simulink model "mix"  (R2018b)
settings: Solver=VariableStepAuto  StartTime=0.0  StopTime=10  RelTol=1e-3
values from neighbouring files (symbols this model uses):
  A = [0,1,0,0;-ks/Il,-cl/Il,ks/Il,0;0,0,0,1;ks/Im,0,-ks/Im,-cm/Im]    [base_mix.m]    (also in optimal_control.m)
  B = [0,0;0,1/Il;0,0;K/Im,0]    [base_mix.m]    (also in optimal_control.m)
  C = [0,0,1,0;1,0,0,0;-ks,0,ks,0]    [base_mix.m]    (also in optimal_control.m)
  D = zeros(3,2)    [base_mix.m]    (also in optimal_control.m)
  G = G(4)    [base_mix.m]    (also in optimal_control.m)
  Kd = (2*ksai_torque*wn_torque+beta_torque)/den    [base_mix.m]
  Kf = acker(A,B(:,1),Target_Pole)    [base_mix.m]    (also in optimal_control.m = lqr(A,B(:,1),Q,R))
  Ki = (beta_torque*wn_torque^2)/den    [base_mix.m]
  Kp = ((2*ksai_torque*wn_torque*beta_torque+wn_torque^2-(Il+Im)*ks/Il/Im))/den    [base_mix.m]
libraries: cstblocks x2, simulink x1
settings Model: Creator=78224  LastModifiedBy=78224

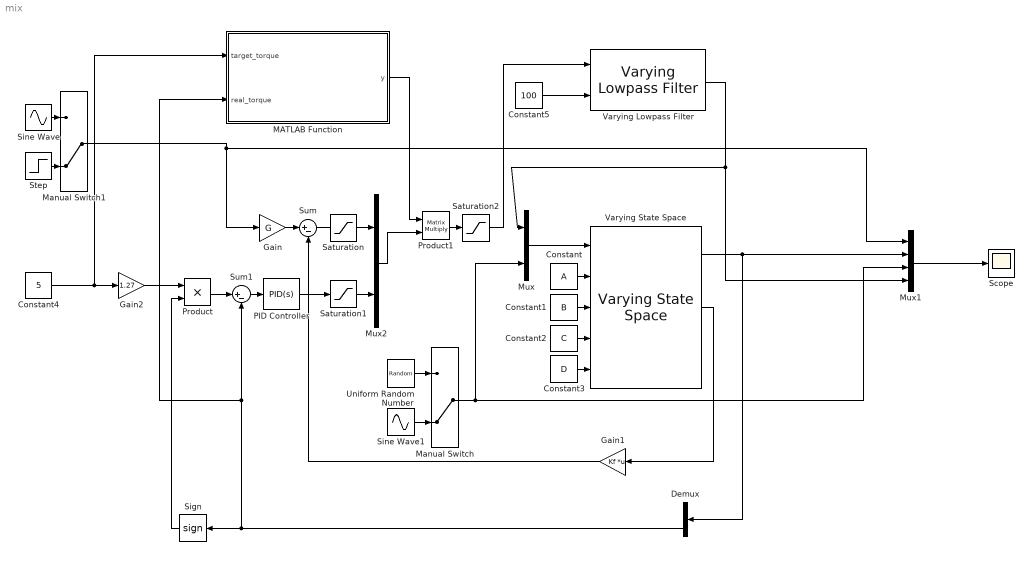
== system mix ==
  Constant : Constant  Value=A  VectorParams1D=off
  Constant1 : Constant  Value=B  VectorParams1D=off
  Constant2 : Constant  Value=C  VectorParams1D=off
  Constant3 : Constant  Value=D  VectorParams1D=off
  Constant4 : Constant  Value=5
  Constant5 : Constant  Value=100
  Demux : Demux  Outputs=3
  Gain : Gain  Gain=G
  Gain1 : Gain  Gain=Kf  Multiplication=Matrix(K*u)
  Gain2 : Gain  Gain=1.27
  MATLAB Function : MATLAB Function  TreatAsAtomicUnit=on
  Manual Switch : ManualSwitch  CurrentSetting=0
  Manual Switch1 : ManualSwitch  CurrentSetting=0
  Mux : Mux  Inputs=2
  Mux1 : Mux
  Mux2 : Mux  Inputs=2
  PID Controller : simulink/Continuous/PID Controller  Controller=PID  Form=Parallel  TimeDomain=Continuous-time  SampleTime=-1  IntegratorMethod=Forward Euler  FilterMethod=Forward Euler  ControllerParametersSource=internal  P=Kp  I=Ki  D=Kd  UseFilter=on  N=100  TunerSelectOption=Transfer Function Based (PID Tuner App)  InitialConditionSource=internal  InitialConditionForIntegrator=0  InitialConditionForFilter=0  DifferentiatorICPrevScaledInput=0  ExternalReset=none  TrackingMode=off  Kt=1  LimitOutput=off  UpperSaturationLimit=inf  LowerSaturationLimit=-inf  LinearizeAsGain=on  AntiWindupMode=none  Kb=1  POutMin=[]  POutMax=[]  IOutMin=[]  IOutMax=[]  DOutMin=[]  DOutMax=[]  NOutMin=[]  NOutMax=[]  SumOutMin=[]  SumOutMax=[]  SaturationOutMin=[]  SaturationOutMax=[]  PParamMin=[]  PParamMax=[]  IParamMin=[]  IParamMax=[]  DParamMin=[]  DParamMax=[]  NParamMin=[]  NParamMax=[]  KbParamMin=[]  KbParamMax=[]  KtParamMin=[]  KtParamMax=[]  KbOutMin=[]  KbOutMax=[]  KtOutMin=[]  KtOutMax=[]  IntegratorOutMin=[]  IntegratorOutMax=[]  FilterOutMin=[]  FilterOutMax=[]  SumI1OutMin=[]  SumI1OutMax=[]  SumI2OutMin=[]  SumI2OutMax=[]  SumI3OutMin=[]  SumI3OutMax=[]  SumI4OutMin=[]  SumI4OutMax=[]  SumDOutMin=[]  SumDOutMax=[]  DifferentiatorOutMin=[]  DifferentiatorOutMax=[]  FilterDiffOutCoefMin=[]  FilterDiffOutCoefMax=[]  ReciprocalOutMin=[]  ReciprocalOutMax=[]  SumDenOutMin=[]  SumDenOutMax=[]  SumNumOutMin=[]  SumNumOutMax=[]  DivideOutMin=[]  DivideOutMax=[]  IntegratorContinuousStateAttributes=''  IntegratorStateMustResolveToSignalObject=off  IntegratorRTWStateStorageClass=Auto  FilterContinuousStateAttributes=''  FilterStateMustResolveToSignalObject=off  FilterRTWStateStorageClass=Auto  ParallelPVariant=InternalParameters  IdealPVariant=Disabled  IVariant=InternalParameters  DVariant=InternalParameters  IntegratorVariant=Continuous  SatVariant=Disabled  AWVariant=Passthrough  PCopyVariant=Disabled  TRVariant=Disabled  FdbkBlocksVariant=Forward  IdealPFdbkVariant=Disabled  SatFdbkVariant=Disabled  DerivativeFilterVariant=ContFilter  NVariant=InternalParameters  NCopyVariant=Disabled  FilterICVariant=InternalICsFilter  IntegratorICVariant=InternalICs  ExternalResetVariant=Disabled  TRSumVariant=Passthrough  SumFdbkVariant=Disabled  SumVariant=Sum_PID
  Product : Product
  Product1 : Product  Multiplication=Matrix(*)
  Saturation : Saturate  UpperLimit=3.12  LowerLimit=-3.12
  Saturation1 : Saturate  UpperLimit=3.12  LowerLimit=-3.12
  Saturation2 : Saturate  UpperLimit=3.12  LowerLimit=-3.12
  Scope : Scope
  Sign : Signum
  Sine Wave : Sin  Amplitude=60  Frequency=2*pi*0.2  SampleTime=0
  Sine Wave1 : Sin  Amplitude=0  Frequency=2*pi*0.2  SampleTime=0
  Step : Step  After=60  SampleTime=0
  Sum : Sum  Inputs=|+-
  Sum1 : Sum  Inputs=|+-
  Uniform Random Number : UniformRandomNumber  Minimum=-5  Maximum=5  SampleTime=0.1
  Varying Lowpass Filter : cstblocks/Linear Parameter Varying/Varying Lowpass Filter  N=1
      settings: SourceProductName=Control System Toolbox
  Varying State Space : cstblocks/Linear Parameter Varying/Varying State Space  x0=0  xNames=''  OutputX=on  OutputDX=on
      settings: SourceProductName=Control System Toolbox
  wires:
  Saturation1/1 -> Mux2/2
  Varying Lowpass Filter/1 -> Mux1/4, Mux/1
  Mux2/1 -> Product1/2
  Step/1 -> Manual Switch1/2
  Sum/1 -> Mux2/1
  PID Controller/1 -> Saturation1/1
  Mux/1 -> Varying State Space/1
  Gain1/1 -> Sum/2
  Constant3/1 -> Varying State Space/5
  Constant4/1 -> Gain2/1, MATLAB Function/1(target_torque)
  Demux/3 -> Sign/1, Sum1/2, MATLAB Function/2(real_torque)
  Constant/1 -> Varying State Space/2
  Gain/1 -> Sum/1
  Varying State Space/2 -> Gain1/1
  Saturation2/1 -> Varying Lowpass Filter/1
  Constant1/1 -> Varying State Space/3
  Manual Switch/1 -> Mux1/3, Mux/2
  Constant2/1 -> Varying State Space/4
  MATLAB Function/1(y) -> Product1/1
  Uniform Random Number/1 -> Manual Switch/1
  Product1/1 -> Saturation2/1
  Sum1/1 -> PID Controller/1
  Sign/1 -> Product/2
  Sine Wave1/1 -> Manual Switch/2
  Constant5/1 -> Varying Lowpass Filter/2
  Manual Switch1/1 -> Gain/1, Mux1/1
  Product/1 -> Sum1/1
  Varying State Space/1 -> Demux/1, Mux1/2
  Sine Wave/1 -> Manual Switch1/1
  Mux1/1 -> Scope/1
  Gain2/1 -> Product/1

== matlab function mix/MATLAB Function ==
  data: y output; target_torque input; real_torque input
function y = evaluate(target_torque, real_torque)
target_torque = target_torque*1;
h = real_torque^2-target_torque^2;
k = 0.05;
w = 1-((min(0,(min(0,h))^4-((k*target_torque)^2-target_torque^2)^4))^4)/((k*target_torque)^2-target_torque^2)^16;

y = [w, 1-w];
